simulink model "Eg7_9"  (R2018a)
settings: Solver=VariableStepAuto  StartTime=0.0  StopTime=10.0  RelTol=1e-3
settings Model: Creator=wangluo  LastModifiedBy=wangluo

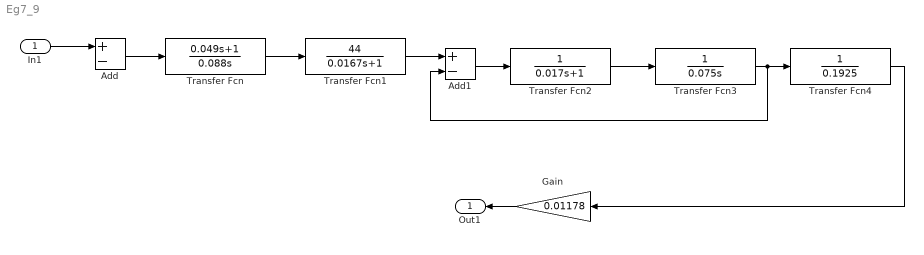
== system Eg7_9 ==
  In1 : Inport
  Add : Sum  Inputs=+-
  Add1 : Sum  Inputs=+-
  Gain : Gain  Gain=0.01178
  Transfer Fcn : TransferFcn  Numerator=[0.049 1]  Denominator=[0.088 0]
  Transfer Fcn1 : TransferFcn  Numerator=[44]  Denominator=[0.0167 1]
  Transfer Fcn2 : TransferFcn  Denominator=[0.017 1]
  Transfer Fcn3 : TransferFcn  Denominator=[0.075 0]
  Transfer Fcn4 : TransferFcn  Denominator=[0.1925]
  Out1 : Outport
  wires:
  In1/1 -> Add/1
  Add/1 -> Transfer Fcn/1
  Transfer Fcn/1 -> Transfer Fcn1/1
  Transfer Fcn1/1 -> Add1/1
  Add1/1 -> Transfer Fcn2/1
  Transfer Fcn2/1 -> Transfer Fcn3/1
  Gain/1 -> Out1/1
  Transfer Fcn3/1 -> Add1/2, Transfer Fcn4/1
  Transfer Fcn4/1 -> Gain/1
